simulink model "Cable_iDesignMask"  (R2020b)
settings: Solver=FixedStepAuto  StartTime=0.0  StopTime=25  RelTol=1e-3
libraries: simulink x1
settings Model: Creator=mebell  LastModifiedBy=nbutler2
settings DataIOCC: ReturnWorkspaceOutputs=off
settings DebuggingCC: ArithmeticOperatorsInVariantConditions=warning
settings SFSimCC: SimUseLocalCustomCode=off  CustomCodeUndefinedFunction=UseInterfaceOnly
settings RTWCC: RTWUseLocalCustomCode=off

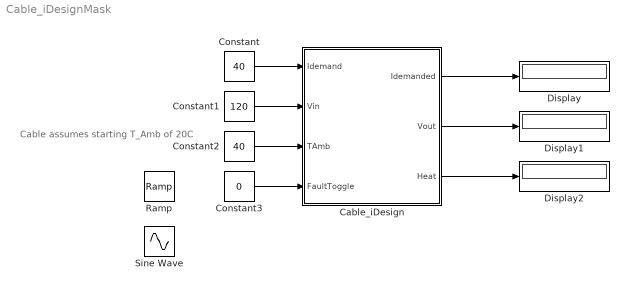
== system Cable_iDesignMask ==
  note: Cable assumes starting T_Amb of 20C
  Cable_iDesign : Subsystem  TreatAsAtomicUnit=on  mask{rad_c_M=0.29854, t_i_M=1.0423, Mass_M=112.1037, R_init=0.06, alpha=0.00393, V_in=120, V_drop=3, I_out=40, Len=100, Mat_c=Copper, Mat_i=PVC, FS=1.5}
      mask prompts: rad_c_M "Conductor Radius [mm]"; t_i_M "Insulator Thickness [mm]"; Mass_M "Mass [g]"; R_init "Resistance at 20C [Ohm]"; V_in "Max Voltage Input [V]"; V_drop "Allowable Voltage Drop [%]"; I_out "Max Current Output [A]"; Len "Desired Cable Length [cm]"; Mat_c "Conductor Material"; Mat_i "Insulator Material"; FS "Factor of Safety"
      mask init:
      | %Get current block name
      | block = gcb;
      | 
      | %Block under the mask(T_in inport and outport)
      | %block2 = [block '/T_in'];
      | 
      | %Set T_in unit parameter to correct unit.
      | %{
      | switch TempIn
      |     case 1 
      |         set_param(block2,'Unit','degF');
      |     case 2
      |         set_param(block2,'Unit','degC');
      |     case 3
      |         set_param(block2,'Unit','degR');
      |     case 4
      |         set_param(block2,'Unit','K');
      | end
      | %}
      mask TypeOptions Mat_c: Copper | Aluminum | Steel
      mask TypeOptions Mat_i: PVC | PE | ETFE
      mask DialogControl Container4 Prompt: Parameters
      mask DialogControl Container5 Prompt: iDesign
      mask DialogControl Container7 Prompt: New Design
      mask DialogControl runButton Prompt: RUN iDESIGN
      mask DialogControl runButton Callback:
      | %Get block handle:
      | blockHandle = getSimulinkBlockHandle(gcb);
      | 
      | %Get values of parameters and convert from string type to numeric data type:
      | V_in = str2num(get_param(blockHandle, 'V_in'));
      | V_drop = str2num(get_param(blockHandle, 'V_drop'));
      | I_out = str2num(get_param(blockHandle, 'I_out'));
      | Length = str2num(get_param(blockHandle, 'Len'));
      | Mat_c = get_param(blockHandle, 'Mat_c');
      | Mat_i = get_param(blockHandle, 'Mat_i');
      | Derat_Fact = str2num(get_param(blockHandle, 'FS'));
      | 
      | %Call iDesign_Cable.m to calculate component values
      | %based on specified operating conditions:
      | 
      | [radius_c, t_i, Mass, R_c, alpha] = iDesign_Cable(V_in, V_drop,...
      |     I_out, Length, Mat_c, Mat_i, Derat_Fact);
      | 
      | %Convert numeric data types to strings so set_param
      | %can assign them to the simulation:
      | radius_c = num2str(radius_c);
      | t_i = num2str(t_i);
      | Mass = num2str(Mass);
      | R_init = num2str(R_c);
      | alpha = num2str(alpha);
      | 
      | %Set block parameters according to the values returned above:
      | set_param(blockHandle, 'rad_c_M', radius_c);
      | set_param(blockHandle, 't_i_M', t_i);
      | set_param(blockHandle, 'Mass_M', Mass);
      | set_param(blockHandle, 'R_init', R_init);
      | set_param(blockHandle, 'alpha', alpha);
      mask Display:
      | port_label('input', 1, 'I_demand');
      | port_label('input', 2, 'Vin');
      | port_label('input', 3, 'TAmb');
      | port_label('input', 4, 'FaultToggle');
      | 
      | port_label('output', 1, 'I_demanded');
      | port_label('output', 2, 'VOut');
      | port_label('output', 3, 'Heat');
  Constant : Constant  Value=40
  Constant1 : Constant  Value=120
  Constant2 : Constant  Value=40
  Constant3 : Constant  Value=0
  Display : Display
  Display1 : Display
  Display2 : Display
  Ramp : simulink/Sources/Ramp  slope=.5  start=5  InitialOutput=20
  Sine Wave : Sin  Amplitude=5  Bias=20  Frequency=.25  SampleTime=0
  wires:
  Constant/1 -> Cable_iDesign/1(Idemand)
  Constant1/1 -> Cable_iDesign/2(Vin)
  Constant2/1 -> Cable_iDesign/3(TAmb)
  Cable_iDesign/1(Idemanded) -> Display/1
  Cable_iDesign/2(Vout) -> Display1/1
  Cable_iDesign/3(Heat) -> Display2/1
  Constant3/1 -> Cable_iDesign/4(FaultToggle)

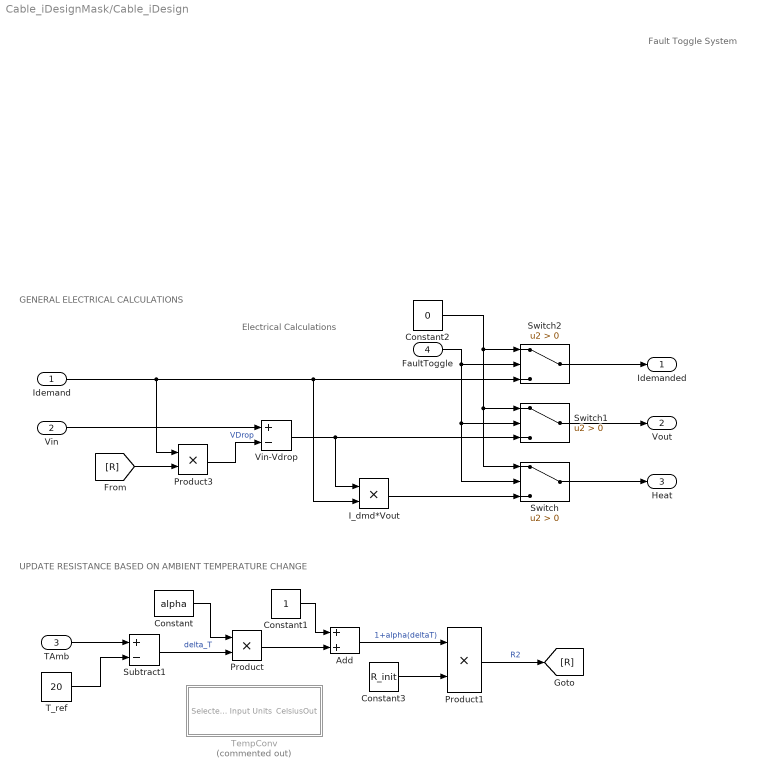
== system Cable_iDesignMask/Cable_iDesign ==
  note: Electrical Calculations
  note: Fault Toggle System
  note: UPDATE RESISTANCE BASED ON AMBIENT TEMPERATURE CHANGE
  note: GENERAL ELECTRICAL CALCULATIONS
  Idemand : Inport
  Vin : Inport  Port=2
  TAmb : Inport  Port=3
  FaultToggle : Inport  Port=4
  Add : Sum
  Constant : Constant  Value=alpha
  Constant1 : Constant
  Constant2 : Constant  Value=0
  Constant3 : Constant  Value=R_init
  I_dmd*Vout : Product
  Product : Product
  Product1 : Product
  Product3 : Product
  Subtract1 : Sum  Inputs=+-
  Switch : Switch  Criteria=u2 > Threshold
  Switch1 : Switch  Criteria=u2 > Threshold
  Switch2 : Switch  Criteria=u2 > Threshold
  T_ref : Constant  Value=20
  TempConv : Subsystem  Commented=on
      mask DialogControl DescTextVar Prompt: Temperature Unit Converter
  Vin-Vdrop : Sum  Inputs=+-
  Idemanded : Outport  VectorParamsAs1DForOutWhenUnconnected=off
  Vout : Outport  Port=2  VectorParamsAs1DForOutWhenUnconnected=off
  Heat : Outport  Port=3  VectorParamsAs1DForOutWhenUnconnected=off
  wires:
  Vin/1 -> Vin-Vdrop/1
  Subtract1/1 -> Product/2  "delta_T"
  Constant/1 -> Product/1
  Product/1 -> Add/2
  Constant1/1 -> Add/1
  Add/1 -> Product1/1  "1+alpha(deltaT)"
  Product1/1 -> [R]  "R2"
  Constant3/1 -> Product1/2
  T_ref/1 -> Subtract1/2
  Vin-Vdrop/1 -> I_dmd*Vout/1, Switch1/3
  Idemand/1 -> Product3/1, I_dmd*Vout/2, Switch2/3
  [R] -> Product3/2
  Product3/1 -> Vin-Vdrop/2  "VDrop"
  Switch1/1 -> Vout/1
  Switch2/1 -> Idemanded/1
  I_dmd*Vout/1 -> Switch/3
  Switch/1 -> Heat/1
  Constant2/1 -> Switch2/1, Switch/1, Switch1/1
  FaultToggle/1 -> Switch1/2, Switch/2, Switch2/2
  TAmb/1 -> Subtract1/1

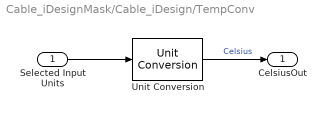
== system Cable_iDesignMask/Cable_iDesign/TempConv ==
  Selected Input Units : Inport
  Unit Conversion : UnitConversion
  CelsiusOut : Outport  Unit=°C  VectorParamsAs1DForOutWhenUnconnected=off
  wires:
  Unit Conversion/1 -> CelsiusOut/1  "Celsius"
  Selected Input Units/1 -> Unit Conversion/1
